simulink model "boostconverter"  (R2019b)
settings: Solver=VariableStepAuto  StartTime=0.0  StopTime=1  RelTol=1e-3
libraries: powerlib x19
settings Model: Creator=q  LastModifiedBy=LENOVO
settings SolverCC: ZeroCrossAlgorithm=Adaptive  AlgebraicLoopSolver=LineSearch
settings DataIOCC: ReturnWorkspaceOutputs=off
settings DebuggingCC: AlgebraicLoopMsg=none  ArtificialAlgebraicLoopMsg=none  IgnoredZcDiagnostic=none  ArithmeticOperatorsInVariantConditions=warning
settings SFSimCC: CustomCodeUndefinedFunction=UseInterfaceOnly

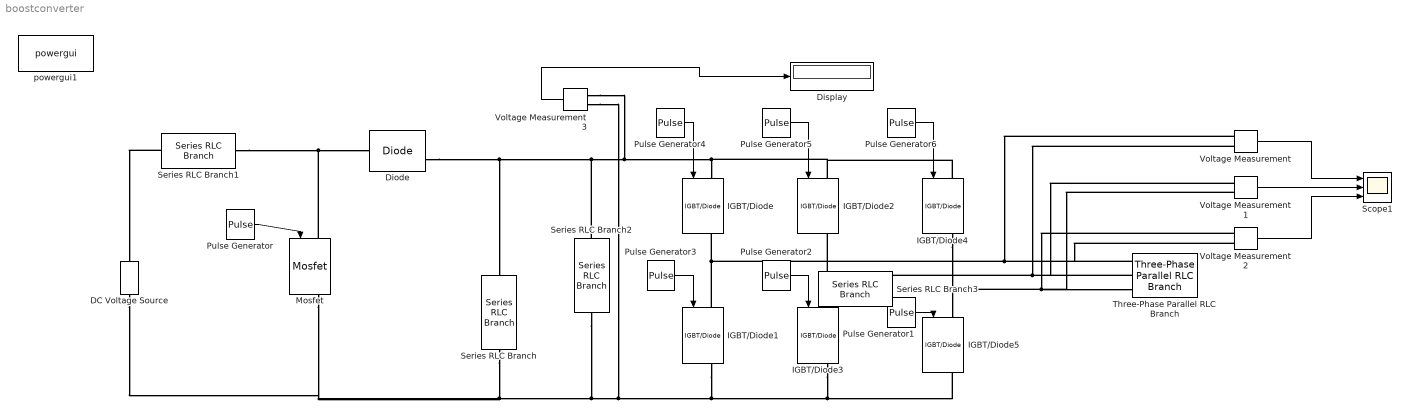
== system boostconverter ==
  DC Voltage Source : powerlib/Electrical Sources/DC Voltage Source  Amplitude=150  Measurements=None
      settings: SourceProductName=Simscape Electrical
  Diode : powerlib/Power Electronics/Diode  Ron=0.001  Lon=0  Vf=0.8  IC=0  UseSnubber=0  Rs=500  Cs=250e-9  Measurements=on
      settings: SourceProductName=Simscape Electrical
  Display : Display
  IGBT/Diode{,1..5} (6 alike) : powerlib/Power Electronics/IGBT//Diode  Ron=1e-3  Rs=1e5  Cs=inf  Measurements=on
      settings: SourceProductName=Simscape Electrical
  Mosfet : powerlib/Power Electronics/Mosfet  Ron=0.001  Lon=0  Rd=0.001  Vfd=0  IC=0  Rs=1e5  Cs=inf  Measurements=on
      settings: SourceProductName=Simscape Electrical
  Pulse Generator : DiscretePulseGenerator  PulseType=Time based  Amplitude=15  Period=0.0002  PulseWidth=50
  Pulse Generator1 : DiscretePulseGenerator  PulseType=Time based  Amplitude=15  Period=0.02  PulseWidth=50  PhaseDelay=0.02*60/360
  Pulse Generator2 : DiscretePulseGenerator  PulseType=Time based  Amplitude=15  Period=0.02  PulseWidth=50  PhaseDelay=0.02*300/360
  Pulse Generator3 : DiscretePulseGenerator  PulseType=Time based  Amplitude=15  Period=0.02  PulseWidth=50  PhaseDelay=0.02*180/360
  Pulse Generator4 : DiscretePulseGenerator  PulseType=Time based  Amplitude=15  Period=0.02  PulseWidth=50
  Pulse Generator5 : DiscretePulseGenerator  PulseType=Time based  Amplitude=15  Period=0.02  PulseWidth=50  PhaseDelay=0.02*120/360
  Pulse Generator6 : DiscretePulseGenerator  PulseType=Time based  Amplitude=15  Period=0.02  PulseWidth=50  PhaseDelay=0.02*240/360
  Scope1 : Scope  NumInputPorts=3
  Series RLC Branch : powerlib/Elements/Series RLC Branch  LConnTagsString=__new0  RConnTagsString=__new0  BranchType=C  Resistance=1  Inductance=1e-3  SetiL0=off  InitialCurrent=0  Capacitance=1e-6  Setx0=off  InitialVoltage=0  Measurements=None
      settings: SourceProductName=Simscape Electrical
  Series RLC Branch1 : powerlib/Elements/Series RLC Branch  LConnTagsString=__new0  RConnTagsString=__new0  BranchType=L  Resistance=1  Inductance=500e-3  SetiL0=off  InitialCurrent=0  Capacitance=1e-6  Setx0=off  InitialVoltage=0  Measurements=None
      settings: SourceProductName=Simscape Electrical
  Series RLC Branch2 : powerlib/Elements/Series RLC Branch  LConnTagsString=__new0  RConnTagsString=__new0  BranchType=R  Resistance=85  Inductance=1e-3  SetiL0=off  InitialCurrent=0  Capacitance=1e-6  Setx0=off  InitialVoltage=0  Measurements=None
      settings: SourceProductName=Simscape Electrical
  Series RLC Branch3 : powerlib/Elements/Series RLC Branch  LConnTagsString=__new0  RConnTagsString=__new0  BranchType=RLC  Resistance=1  Inductance=1e-3  SetiL0=off  InitialCurrent=0  Capacitance=1e-6  Setx0=off  InitialVoltage=0  Measurements=None
      settings: SourceProductName=Simscape Electrical
  Three-Phase Parallel RLC Branch : powerlib/Elements/Three-Phase Parallel RLC Branch  LConnTagsString=A|B|C  RConnTagsString=A|B|C  BranchType=RLC  Resistance=1  Inductance=1e-3  Capacitance=1e-6  Measurements=None
      settings: SourceProductName=Simscape Electrical  SourceProductBaseCode=PS
  Voltage Measurement{,1..3} (4 alike) : powerlib/Measurements/Voltage Measurement  PhasorSimulation=off  OutputType=Complex  PSBequivalent=0
      settings: SourceProductName=Simscape Electrical
  powergui1 : powerlib/powergui  Priority=1  SimulationMode=Continuous  SampleTime=50e-6  frequency=60  Iterations=50  frequencyindice=0  Pbase=100e6  ErrMax=1e-4  UnitsV=kV  UnitsW=MW  buscounter=0  FunctionMessages=off  echomessages=off  EnableUseOfTLC=off  CurrentSourceSwitches=off  DisableSnubberDevices=off  DisableRonSwitches=off  DisableVfSwitches=off  DisplayEquations=off  AutomaticDiscreteSolvers=off  SolverType=Tustin/Backward Euler (TBE)  Interpol=off  ExternalGateDelay=off  methode=off  Ts=100  x0status=blocks  SPID=on  SwTol=0  HookPort=off  NonlinearTolerance=1e-4  nMaxIteration=100  ContinueOnMaxIteration=off  RestoreLinks=warning  ResistiveCurrentMeasurement=off  Frange=[0:2:500]  Ylog=off  Xlog=on  ShowGrid=off  save=off  variable=ZData  structure=0  ZoomFFT=off  StartTime=0.0  cycles=1  DisplayStyle=1  fundamental=60  FreqAxis=off  MaxFrequency=1000  frequencyindicesteady=1  RmsSteady=1  display=off
      settings: SourceProductName=Simscape Electrical
  wires:
  Pulse Generator/1 -> Mosfet/1
  Pulse Generator1/1 -> IGBT/Diode5/1
  Pulse Generator2/1 -> IGBT/Diode3/1
  Pulse Generator3/1 -> IGBT/Diode1/1
  Pulse Generator4/1 -> IGBT/Diode/1
  Pulse Generator5/1 -> IGBT/Diode2/1
  Pulse Generator6/1 -> IGBT/Diode4/1
  Voltage Measurement/1 -> Scope1/1
  Voltage Measurement1/1 -> Scope1/2
  Voltage Measurement2/1 -> Scope1/3
  Voltage Measurement3/1 -> Display/1
  connections:
  Series RLC Branch1/RConn1 -- Diode/LConn1 -- Mosfet/LConn1
  IGBT/Diode1/LConn1 -- Voltage Measurement/LConn1 -- Three-Phase Parallel RLC Branch/LConn1 -- Voltage Measurement2/LConn2 -- IGBT/Diode/RConn1
  IGBT/Diode3/LConn1 -- Three-Phase Parallel RLC Branch/LConn2 -- Voltage Measurement1/LConn1 -- Voltage Measurement/LConn2 -- IGBT/Diode2/RConn1
  IGBT/Diode4/RConn1 -- Voltage Measurement2/LConn1 -- Three-Phase Parallel RLC Branch/LConn3 -- Voltage Measurement1/LConn2 -- IGBT/Diode5/LConn1
  Diode/RConn1 -- Series RLC Branch/RConn1 -- Voltage Measurement3/LConn1 -- IGBT/Diode4/LConn1 -- IGBT/Diode2/LConn1 -- IGBT/Diode/LConn1 -- Series RLC Branch2/LConn1
  Series RLC Branch/LConn1 -- DC Voltage Source/LConn1 -- Mosfet/RConn1 -- Series RLC Branch2/RConn1 -- Voltage Measurement3/LConn2 -- IGBT/Diode1/RConn1 -- IGBT/Diode5/RConn1 -- IGBT/Diode3/RConn1
  Series RLC Branch1/LConn1 -- DC Voltage Source/RConn1
